simulink model "asbCubeSatArchModel"  (R2024b)
settings: configuration reference "CubeSatConfigSet" (kept outside this file)
InitFcn:
  | detectChangeOrbitalElements;
(part 2 of 2)

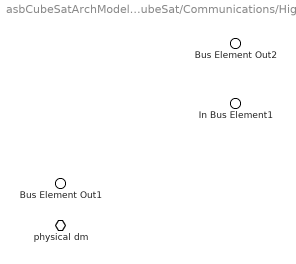
== system asbCubeSatArchModel/CubeSat Mission Enterprise/Space Segment/CubeSat/Communications/High Rate Antenna ==
  In Bus Element1 : Inport  PortName=hr encoded xmit
  physical dm : PMIOPort  Side=Right
  Bus Element Out2 : Outport  PortName=orientation data
  Bus Element Out1 : Outport  Port=2  PortName=observation data RF

== system asbCubeSatArchModel/CubeSat Mission Enterprise/Space Segment/CubeSat/Communications/LR Xmit Amplifier ==
  In Bus Element1 : Inport  PortName=lr encode
  Bus Element Out1 : Outport  PortName=lr encoded xmit 2

== system asbCubeSatArchModel/CubeSat Mission Enterprise/Space Segment/CubeSat/Communications/Low Rate Antenna ==
  Bus Element In2 : Inport  PortName=encoded xmit 2
  Bus Element In1 : Inport  Port=2  PortName=gnd cmd
  Bus Element Out2 : Outport  PortName=lr xmit
  Bus Element Out1 : Outport  Port=2  PortName=telemetry

== system asbCubeSatArchModel/CubeSat Mission Enterprise/Space Segment/CubeSat/Communications/RF Rcvr-Decoder ==
  Bus Element In1 : Inport  PortName=lr recv
  Bus Element Out1 : Outport  PortName=cmd

== system asbCubeSatArchModel/CubeSat Mission Enterprise/Space Segment/CubeSat/Communications/RF Xmit-Encoder ==
  In Bus Element1 : Inport  PortName=tlm data
  In Bus Element2 : Inport  Port=2  PortName=mission data 2
  Out Bus Element1 : Outport  PortName=lr encode
  Out Bus Element2 : Outport  Port=2  PortName=hr encode

== system asbCubeSatArchModel/CubeSat Mission Enterprise/Space Segment/CubeSat/GNC/Adapter ==
  In Bus Element : Inport  PortName=Environment
  Out Bus Element : Outport  PortName=Out
  wires:
  In Bus Element/1 -> Out Bus Element/1

== system asbCubeSatArchModel/CubeSat Mission Enterprise/Space Segment/CubeSat/GNC/Adapter1 ==
  In Bus Element : Inport  PortName=SensorsOut
  Out Bus Element : Outport  PortName=Input
  wires:
  In Bus Element/1 -> Out Bus Element/1

== system asbCubeSatArchModel/CubeSat Mission Enterprise/Space Segment/CubeSat/Power/Power System Control ==
  Bus Element In2 : Inport  PortName=attitudeStates
  Bus Element In1 : Inport  Port=2  PortName=sensorData
  Bus Element Out1 : Outport  PortName=actuatorCmd

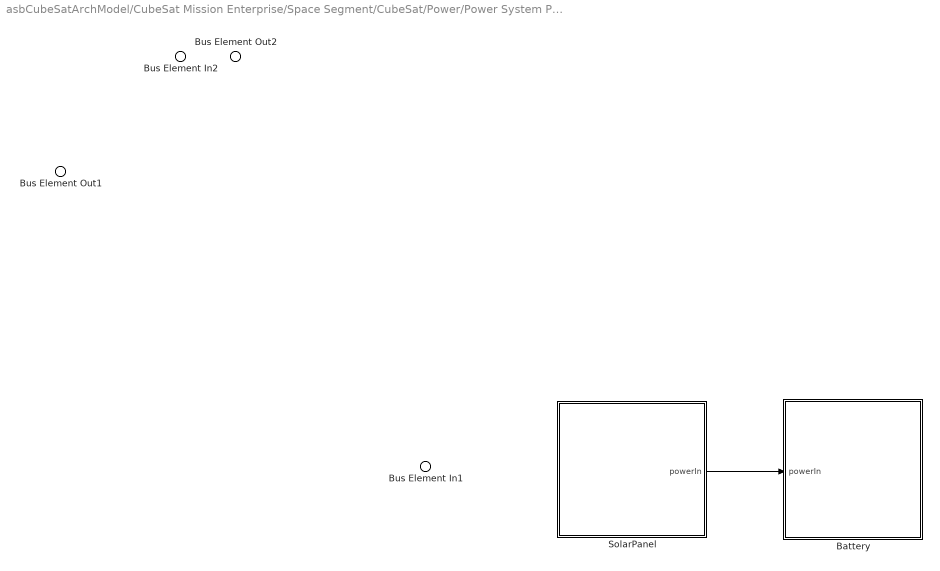
== system asbCubeSatArchModel/CubeSat Mission Enterprise/Space Segment/CubeSat/Power/Power System Plant ==
  Bus Element In2 : Inport  PortName=attitudeStates
  Bus Element In1 : Inport  Port=2  PortName=actuatorCmd
  Battery : Subsystem
      settings: PortSchema="{\"entries\":[{\"content\":{\"headerSize\":26,\"margin\":15,\"minimumSpacing\":25,\"sides\":[{\"content\":{\"connectorIds\":[\"In1\"]},\"type\":\"ConnectorPlacement.EquallySpacedRectSide\",\"uuid\":\"99007498-99ba-4c23-a0a0-87e1543943ee\"},{\"content\":{\"connectorIds\":[],\"side\":\"RIGHT\"},\"type\":\"ConnectorPlacement.EquallySpacedRectSide\",\"uuid\":\"554f3d31-4e95-4b23-9d3b-85f383ee0045\"},{\"content\":{\"connectorIds\":[],\"side\":\"TOP\"},\"type\":\"ConnectorPlacement.EquallySpacedRectSide\",\"uuid\":\"16cf11e7-d1a7-4edd-b8c5-05af2e73c5bd\"}]},\"type\":\"ConnectorPlacement.EquallySpacedConnector\",\"uuid\":\"0a651afa-d7fb-4b32-a21c-81d6f3c917ae\"}],\"packageUris\":[\"http://schema.mathworks.com/mf0/Connector/R2020b\"],\"version\":\"1.0\"}"
  SolarPanel : Subsystem  RequirementInfo="{}  %GIDa_4f725f0c_e8f4_4f8d_a212_700d35e9a783"
      settings: PortSchema="{\"entries\":[{\"content\":{\"headerSize\":26,\"margin\":15,\"minimumSpacing\":25,\"sides\":[{\"content\":{\"connectorIds\":[]},\"type\":\"ConnectorPlacement.EquallySpacedRectSide\",\"uuid\":\"bdb7f036-cfc5-488a-888f-b9d18995973e\"},{\"content\":{\"connectorIds\":[\"Out1\"],\"side\":\"RIGHT\"},\"type\":\"ConnectorPlacement.EquallySpacedRectSide\",\"uuid\":\"bf580f20-7193-4743-ad48-17eb92535429\"},{\"content\":{\"connectorIds\":[],\"side\":\"TOP\"},\"type\":\"ConnectorPlacement.EquallySpacedRectSide\",\"uuid\":\"da6f3a46-474d-4698-8115-df2cb74be4ae\"}]},\"type\":\"ConnectorPlacement.EquallySpacedConnector\",\"uuid\":\"514a736b-bd6f-43cb-ac87-4eaa6b5005de\"}],\"packageUris\":[\"http://schema.mathworks.com/mf0/Connector/R2020b\"],\"version\":\"1.0\"}"
  Bus Element Out2 : Outport  PortName=powerStates
  Bus Element Out1 : Outport  Port=2  PortName=sensorData
  wires:
  SolarPanel/1(powerIn) -> Battery/1(powerIn)

== system asbCubeSatArchModel/CubeSat Mission Enterprise/Space Segment/CubeSat/Power/Power System Plant/Battery ==
  Bus Element In1 : Inport  PortName=powerIn
  BatteryCell : Subsystem
      settings: PortSchema="{\"entries\":[{\"content\":{\"headerSize\":26,\"margin\":15,\"minimumSpacing\":25,\"sides\":[{\"content\":{\"connectorIds\":[]},\"type\":\"ConnectorPlacement.EquallySpacedRectSide\",\"uuid\":\"bdb7f036-cfc5-488a-888f-b9d18995973e\"},{\"content\":{\"connectorIds\":[],\"side\":\"RIGHT\"},\"type\":\"ConnectorPlacement.EquallySpacedRectSide\",\"uuid\":\"bf580f20-7193-4743-ad48-17eb92535429\"},{\"content\":{\"connectorIds\":[],\"side\":\"TOP\"},\"type\":\"ConnectorPlacement.EquallySpacedRectSide\",\"uuid\":\"da6f3a46-474d-4698-8115-df2cb74be4ae\"}]},\"type\":\"ConnectorPlacement.EquallySpacedConnector\",\"uuid\":\"514a736b-bd6f-43cb-ac87-4eaa6b5005de\"}],\"packageUris\":[\"http://schema.mathworks.com/mf0/Connector/19700101\"],\"version\":\"1.0\"}"

== system asbCubeSatArchModel/CubeSat Mission Enterprise/Space Segment/CubeSat/Power/Power System Plant/SolarPanel ==
  SolarPanelCell : Subsystem
      settings: PortSchema="{\"entries\":[{\"content\":{\"headerSize\":26,\"margin\":15,\"minimumSpacing\":25,\"sides\":[{\"content\":{\"connectorIds\":[]},\"type\":\"ConnectorPlacement.EquallySpacedRectSide\",\"uuid\":\"bdb7f036-cfc5-488a-888f-b9d18995973e\"},{\"content\":{\"connectorIds\":[],\"side\":\"RIGHT\"},\"type\":\"ConnectorPlacement.EquallySpacedRectSide\",\"uuid\":\"bf580f20-7193-4743-ad48-17eb92535429\"},{\"content\":{\"connectorIds\":[],\"side\":\"TOP\"},\"type\":\"ConnectorPlacement.EquallySpacedRectSide\",\"uuid\":\"da6f3a46-474d-4698-8115-df2cb74be4ae\"}]},\"type\":\"ConnectorPlacement.EquallySpacedConnector\",\"uuid\":\"514a736b-bd6f-43cb-ac87-4eaa6b5005de\"}],\"packageUris\":[\"http://schema.mathworks.com/mf0/Connector/19700101\"],\"version\":\"1.0\"}"
  Bus Element Out1 : Outport  PortName=powerIn

== system asbCubeSatArchModel/CubeSat Mission Enterprise/Space Segment/CubeSat/Power/Power System Plant/Battery/BatteryCell ==

== system asbCubeSatArchModel/CubeSat Mission Enterprise/Space Segment/CubeSat/Power/Power System Plant/SolarPanel/SolarPanelCell ==
